simulink model "MAIN_Submitted_to_UMD_V2_PCLC"  (R2024a)
settings: Solver=ode3  StartTime=0.0  StopTime=T_end  FixedStep=0.01  RelTol=1e-3  EnableMultiTasking=on
values from neighbouring files (symbols this model uses):
  A1 = x(1)    [MAIN_Protocol_Simulation.m]    (also in find_fluid_profile.m)
  A2 = x(2)    [MAIN_Protocol_Simulation.m]    (also in find_fluid_profile.m)
  A3 = x(8)    [MAIN_Protocol_Simulation.m]    (also in find_fluid_profile.m)
  A4 = x(12)    [MAIN_Protocol_Simulation.m]    (also in find_fluid_profile.m)
  b_control = T(speed,3)    [MAIN_Protocol_Simulation.m]    (also in find_fluid_profile.m)
  B_Gain = x(3)    [MAIN_Protocol_Simulation.m]    (also in find_fluid_profile.m)
  B_Loss = x(4)    [MAIN_Protocol_Simulation.m]    (also in find_fluid_profile.m)
  BP_Tar = x(14)    [MAIN_Protocol_Simulation.m]    (also in find_fluid_profile.m)
  BV0 = x(25)    [MAIN_Protocol_Simulation.m]    (also in find_fluid_profile.m)
  c_start = VP_Inputs.ind_CL_start*Dt    [MAIN_Protocol_Simulation.m]
  G1 = x(15)    [MAIN_Protocol_Simulation.m]    (also in find_fluid_profile.m)
  G2 = x(16)    [MAIN_Protocol_Simulation.m]    (also in find_fluid_profile.m)
  G3 = x(19)    [MAIN_Protocol_Simulation.m]    (also in find_fluid_profile.m)
  Gsv1 = x(6)    [MAIN_Protocol_Simulation.m]    (also in find_fluid_profile.m)
  Gsv2 = x(7)    [MAIN_Protocol_Simulation.m]    (also in find_fluid_profile.m)
  Hct0 = x(24)    [MAIN_Protocol_Simulation.m]    (also in find_fluid_profile.m)
  HR0 = x(22)    [MAIN_Protocol_Simulation.m]    (also in find_fluid_profile.m)
  Ki4 = x(21)    [MAIN_Protocol_Simulation.m]    (also in find_fluid_profile.m)
  Ki_control = T(speed,2)    [MAIN_Protocol_Simulation.m]    (also in find_fluid_profile.m)
  Kp = x(5)    [MAIN_Protocol_Simulation.m]    (also in find_fluid_profile.m)
  Kp2 = x(10)    [MAIN_Protocol_Simulation.m]    (also in find_fluid_profile.m)
  Kp3 = x(11)    [MAIN_Protocol_Simulation.m]    (also in find_fluid_profile.m)
  Kp4 = x(20)    [MAIN_Protocol_Simulation.m]    (also in find_fluid_profile.m)
  Kp_control = T(speed,1)    [MAIN_Protocol_Simulation.m]    (also in find_fluid_profile.m)
  pow1 = x(17)    [MAIN_Protocol_Simulation.m]    (also in find_fluid_profile.m)
  pow2 = x(18)    [MAIN_Protocol_Simulation.m]    (also in find_fluid_profile.m)
  SV0 = x(23)    [MAIN_Protocol_Simulation.m]    (also in find_fluid_profile.m = theta_s(18))
  SV_Tar = x(9)    [MAIN_Protocol_Simulation.m]    (also in find_fluid_profile.m)
  target = DATASET{1,sidx}.Controller_Target    [MAIN_Protocol_Simulation.m]
  TPR0 = x(13)    [MAIN_Protocol_Simulation.m]    (also in find_fluid_profile.m)
  u_max = 2000    [MAIN_Protocol_Simulation.m]    (also in controller_discrete_time.m; find_fluid_profile.m)
libraries: simulink x3
settings Model: Creator=Ramin  LastModifiedBy=yekanth
settings SolverCC: AlgebraicLoopSolver=TrustRegion
settings DataIOCC: LimitDataPoints=on  SaveFormat=Array  SignalLoggingSaveFormat=ModelDataLogs  ReturnWorkspaceOutputs=off
settings OptimizationCC: ExpressionDepthLimit=2147483647  LifeSpan=inf
settings DebuggingCC: UnderspecifiedInitializationDetection=Classic  MergeDetectMultiDrivingBlocksExec=none  SolverPrmCheckMsg=warning  FcnCallInpInsideContextMsg=warning  UnconnectedInputMsg=warning  UnconnectedOutputMsg=warning  UnconnectedLineMsg=warning  StateNameClashWarn=warning  SFUnexpectedBacktrackingDiag=warning  SFNoUnconditionalDefaultTransitionDiag=warning  SFExecutionAtInitializationDiag=none  ArithmeticOperatorsInVariantConditions=warning
settings HardwareCC: ProdBitPerPointer=32  ProdBitPerSizeT=32  ProdBitPerPtrDiffT=32  ProdLargestAtomicFloat=None  ProdIntDivRoundTo=Undefined  ProdEndianess=Unspecified  ProdWordSize=32  ProdHWDeviceType=32-bit Generic
settings ModelReferenceCC: EnableRefExpFcnMdlSchedulingChecks=on  PropagateSignalLabelsOutOfModel=off
settings SFSimCC: SimUseLocalCustomCode=off  CustomCodeUndefinedFunction=UseInterfaceOnly
settings RTWCC: RTWUseLocalCustomCode=off  GPUComputeCapability=3.5
settings CodeAppCC: StateflowObjectComments=on
settings GRTTargetCC: TargetLangStandard=C89/C90 (ANSI)
settings ConfigComp: CovMetricSettings=dw  CovSaveCumulativeToWorkspaceVar=on  CovSaveSingleToWorkspaceVar=on  CovExternalEMLEnable=off

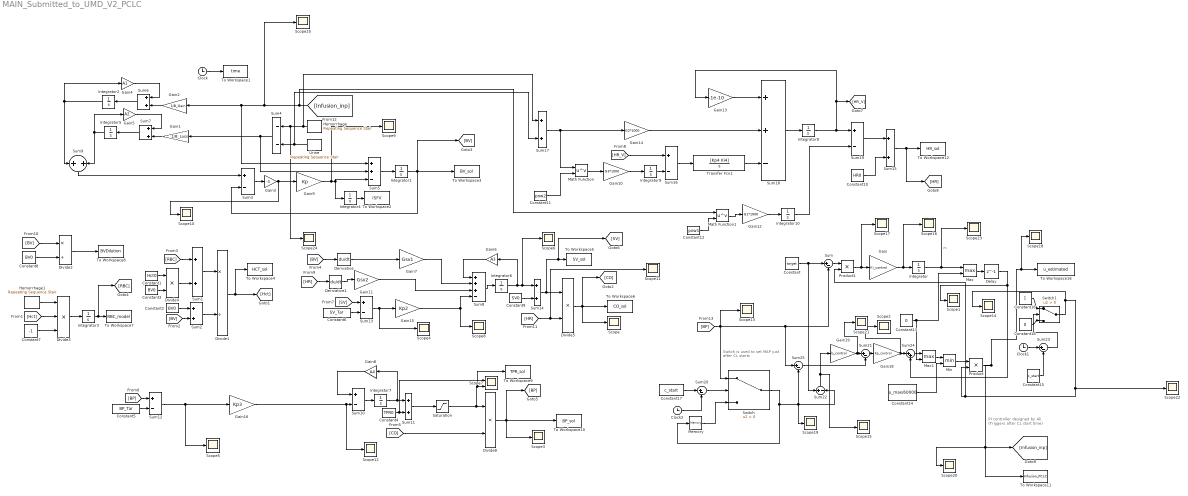
== system MAIN_Submitted_to_UMD_V2_PCLC ==
  note: PI controller designed by Ali
      | (Triggers after CL start time)
  note: Switch is used to set MAP just
      |  after CL starts
  Clock : Clock
  Clock1 : Clock
  Clock2 : Clock
  Constant : Constant  Value=target
  Constant1 : Constant  Value=Hct0
  Constant10 : Constant  Value=HR0
  Constant11 : Constant  Value=pow2
  Constant12 : Constant  Value=pow1
  Constant13 : Constant  Value=0
  Constant14 : Constant  Value=u_max/60000
  Constant15 : Constant  Value=c_start
  Constant16 : Constant
  Constant17 : Constant  Value=c_start
  Constant18 : Constant  Value=0
  Constant2 : Constant  Value=BV0
  Constant3 : Constant  Value=BV0
  Constant4 : Constant  Value=TPR0
  Constant5 : Constant  Value=BP_Tar
  Constant6 : Constant  Value=SV_Tar
  Constant7 : Constant  Value=-1
  Constant8 : Constant  Value=BV0
  Constant9 : Constant  Value=SV0
  Delay : Delay  DelayLength=1  InitialCondition=0
  Derivative : Derivative
  Derivative1 : Derivative
  Divide1 : Product  Inputs=*/
  Divide2 : Product  Inputs=*/
  Divide3 : Product  Inputs=***
  Divide4 : Product  Inputs=**
  Divide5 : Product  Inputs=**
  Divide8 : Product  Inputs=**
  Gain : Gain  Gain=Ki_control
  Gain1 : Gain  Gain=1/B_Loss
  Gain10 : Gain  Gain=G3*1000
  Gain11 : Gain  Gain=Gsv2
  Gain12 : Gain  Gain=G1*1000
  Gain13 : Gain  Gain=-1e-10
  Gain14 : Gain  Gain=G2*1000
  Gain15 : Gain  Gain=Kp2
  Gain16 : Gain  Gain=Kp3
  Gain18 : Gain  Gain=Kp_control
  Gain19 : Gain  Gain=b_control
  Gain2 : Gain  Gain=1/B_Gain
  Gain3 : Gain  Gain=-1
  Gain4 : Gain  Gain=A1
  Gain5 : Gain  Gain=A2
  Gain6 : Gain  Gain=A3
  Gain7 : Gain  Gain=Gsv1
  Gain8 : Gain  Gain=A4
  Gain9 : Gain  Gain=Kp
  Hemorrhage : simulink/Sources/Repeating Sequence Stair  OutValues=Hemorrhage_inp  tsamp=SamplingTime  OutMin=[]  OutMax=[]  OutDataTypeStr=double  OutputDataTypeScalingMode=double  OutDataType=fixdt(0,8)  ConRadixGroup=Best Precision: Vector-wise  OutScaling=2^-12
  Hemorrhage1 : simulink/Sources/Repeating Sequence Stair  OutValues=Hemorrhage_inp  tsamp=SamplingTime  OutMin=[]  OutMax=[]  OutDataTypeStr=double  OutputDataTypeScalingMode=double  OutDataType=fixdt(0,8)  ConRadixGroup=Best Precision: Vector-wise  OutScaling=2^-12
  Integrator{,1..10} (11 alike) : Integrator
  Math Function : Math  Operator=pow  SignedPower=on
  Math Function1 : Math  Operator=pow  SignedPower=on
  Max : MinMax  Function=max  Inputs=2
  Max1 : MinMax  Function=max  Inputs=2
  Memory : Memory
  Min : MinMax  Inputs=2
  Product : Product
  Product1 : Product
  Saturation : Saturate  UpperLimit=4000  LowerLimit=0
  Scope{,1..6,8..25} (25 alike) : Scope
  Scope7 : Scope  NumInputPorts=2
  Sum{,20..21,23,25} (5 alike) : Sum  Inputs=|+-
  Sum{1..2,6..7,9,11,14..15,17} (9 alike) : Sum
  Sum{3,10,12..13,16,19,22} (7 alike) : Sum  Inputs=+-
  Sum18 : Sum  Inputs=++-
  Sum24 : Sum  Inputs=|++
  Sum4 : Sum  Inputs=--
  Sum5 : Sum  Inputs=++-
  Sum8 : Sum  Inputs=+++-
  Switch : Switch  Criteria=u2 > Threshold  SaturateOnIntegerOverflow=off  InputSameDT=off
  Switch1 : Switch  Criteria=u2 > Threshold  SaturateOnIntegerOverflow=off  InputSameDT=off
  To Workspace1 : ToWorkspace  VariableName=time  SampleTime=-1
  To Workspace10 : ToWorkspace  VariableName=BP_sol  SampleTime=-1
  To Workspace11 : ToWorkspace  VariableName=Infusion_PCLC  SampleTime=-1
  To Workspace12 : ToWorkspace  VariableName=HR_sol  SampleTime=-1
  To Workspace16 : ToWorkspace  VariableName=u_estimated  SaveFormat=Timeseries  SampleTime=-1
  To Workspace2 : ToWorkspace  VariableName=ISFV  SampleTime=-1
  To Workspace3 : ToWorkspace  VariableName=BV_sol  SampleTime=-1
  To Workspace4 : ToWorkspace  VariableName=HCT_sol  SampleTime=-1
  To Workspace5 : ToWorkspace  VariableName=SV_sol  SampleTime=-1
  To Workspace6 : ToWorkspace  VariableName=CO_sol  SampleTime=-1
  To Workspace7 : ToWorkspace  VariableName=RBC_model  SampleTime=-1
  To Workspace8 : ToWorkspace  VariableName=BVDilution  SampleTime=-1
  To Workspace9 : ToWorkspace  VariableName=TPR_sol  SampleTime=-1
  Transfer Fcn1 : TransferFcn  Numerator=[Kp4 Ki4]  Denominator=[1 0]
  Urine : simulink/Sources/Repeating Sequence Stair  OutValues=Urine_inp  tsamp=SamplingTime  OutMin=[]  OutMax=[]  OutDataTypeStr=double  OutputDataTypeScalingMode=double  OutDataType=fixdt(0,8)  ConRadixGroup=Best Precision: Vector-wise  OutScaling=2^-12
  wires:
  Integrator4/1 -> To Workspace2/1
  Gain3/1 -> Gain9/1, Scope10/1
  Gain9/1 -> Scope9/1, Sum5/3, Integrator4/1
  Sum3/1 -> Gain3/1
  Sum5/1 -> Integrator1/1
  Divide3/1 -> Integrator3/1
  Integrator3/1 -> [RBC], To Workspace7/1
  Clock/1 -> To Workspace1/1
  [BV] -> Divide2/1
  Constant8/1 -> Divide2/2
  Divide2/1 -> To Workspace8/1
  Hemorrhage1/1 -> Divide3/1
  [Hct] -> Divide3/2
  Sum2/1 -> Divide1/2
  Constant7/1 -> Divide3/3
  Constant2/1 -> Sum2/1
  [BV] -> Sum2/2
  Constant1/1 -> Divide4/1
  Constant3/1 -> Divide4/2
  Divide4/1 -> Sum1/2
  [RBC] -> Sum1/1
  Sum1/1 -> Divide1/1
  Divide1/1 -> [Hct], To Workspace4/1
  Integrator2/1 -> Sum9/1, Gain4/1
  Sum6/1 -> Integrator2/1
  Gain4/1 -> Sum6/1
  Gain2/1 -> Sum6/2
  Integrator5/1 -> Sum9/2, Gain5/1
  Gain1/1 -> Sum7/2
  Sum7/1 -> Integrator5/1
  Gain5/1 -> Sum7/1
  Sum9/1 -> Sum3/1
  Integrator1/1 -> Sum3/2, To Workspace3/1, [BV]
  Gain7/1 -> Sum8/2
  Sum8/1 -> Integrator6/1
  Integrator6/1 -> Sum14/1, Scope6/1, Gain6/1
  Gain6/1 -> Sum8/1
  Constant9/1 -> Sum14/2
  Sum14/1 -> [SV], To Workspace5/1, Divide5/1
  Constant6/1 -> Sum13/2
  Sum13/1 -> Gain15/1, Scope4/1
  [SV] -> Sum13/1
  Gain15/1 -> Scope8/1, Sum8/4
  [BV] -> Derivative/1
  [HR] -> Scope11/1, Divide5/2
  [HR] -> Derivative1/1
  Gain11/1 -> Sum8/3
  Divide5/1 -> [CO], To Workspace6/1, Scope/1
  [BP] -> Sum12/1
  Gain8/1 -> Sum10/1
  Sum11/1 -> Saturation/1
  Sum10/1 -> Integrator7/1
  [CO] -> Divide8/2
  Sum12/1 -> Gain16/1, Scope5/1
  Constant5/1 -> Sum12/2
  Constant4/1 -> Scope7/1, Sum11/2
  Integrator7/1 -> Gain8/1, Sum11/1
  Derivative1/1 -> Gain11/1
  Derivative/1 -> Gain7/1
  Divide8/1 -> To Workspace10/1, Scope3/1, [BP]
  Gain16/1 -> Scope12/1, Sum10/2
  Sum19/1 -> Sum15/1
  [HR_V] -> Sum16/1
  Sum4/1 -> Gain1/1, Sum5/2
  Gain12/1 -> Integrator10/1
  Integrator9/1 -> Sum16/2
  Constant11/1 -> Math Function/2
  Gain13/1 -> Sum18/1
  Math Function1/1 -> Gain12/1
  [Infusion_inp] -> Math Function1/1, Scope25/1, Sum5/1, Gain2/1
  Integrator8/1 -> [HR_V], Gain13/1, Sum19/1
  Hemorrhage/1 -> Scope24/1, Sum4/1, Sum17/1
  Gain14/1 -> Sum18/2
  Constant10/1 -> Sum15/2
  Urine/1 -> Sum17/2, Sum4/2
  Integrator10/1 -> Sum19/2
  Sum15/1 -> [HR], To Workspace12/1
  Math Function/1 -> Gain10/1
  Gain10/1 -> Integrator9/1
  Sum18/1 -> Integrator8/1
  Transfer Fcn1/1 -> Sum18/3
  Sum16/1 -> Transfer Fcn1/1
  Constant12/1 -> Math Function1/2
  Sum17/1 -> Gain14/1, Math Function/1
  Saturation/1 -> To Workspace9/1, Scope7/2, Divide8/1
  Product/1 -> [Infusion_inp], Scope20/1, To Workspace11/1, Scope18/1, To Workspace16/1
  Clock1/1 -> Sum23/1
  Sum23/1 -> Switch1/2
  Sum20/1 -> Switch/2
  Gain/1 -> Integrator/1, Scope16/1
  Constant13/1 -> Max/2, Max1/2
  Switch1/1 -> Scope14/1, Product1/2, Product/2, Scope22/1
  Sum24/1 -> Max1/1
  Integrator/1 -> Scope23/1, Max/1  "m"
  Constant/1 -> Sum/1, Sum22/1
  Constant15/1 -> Sum23/2
  Max1/1 -> Min/1
  Min/1 -> Product/1
  Switch/1 -> Scope19/1, Sum25/2, Sum22/2, Memory/1
  Delay/1 -> Scope1/1, Sum24/2
  Sum22/1 -> Scope15/1, Gain19/1
  Memory/1 -> Switch/3
  Sum21/1 -> Gain18/1
  Constant17/1 -> Sum20/1
  Max/1 -> Delay/1
  [BP] -> Scope13/1, Sum25/1, Sum/2, Switch/1
  Gain19/1 -> Scope21/1, Sum21/1
  Constant14/1 -> Min/2
  Sum25/1 -> Sum21/2
  Clock2/1 -> Sum20/2
  Gain18/1 -> Scope2/1, Sum24/1
  Sum/1 -> Product1/1
  Product1/1 -> Scope17/1, Gain/1
  Constant16/1 -> Switch1/1
  Constant18/1 -> Switch1/3
